simulink model "WF_onshore"  (R2024a)
settings: Solver=VariableStepAuto  StartTime=0  StopTime=0.9  RelTol=1e-3
values from neighbouring files (symbols this model uses):
  cvtr = initialize_NR_VSC_GF(cvtr)    [NR_steadystate_VSC_GF.m]    (also in WF_onshore_SSO_GFL.m = setfield(cvtr,'parameters', p_vary.name,p_vary.val(i)); WF_physical_param_offshore_supersynchronous.m = setfield(cvtr,'parameters', p_vary.name,p_vary.val(i)); WF_physical_param_onshore_SSO_020625.m = setfield(cvtr,'parameters', p_vary.name,p_vary.val(i)); impedance_WT_blackbox.m = base_values(cvtr))
  cvtr1 = cvtr_agg    [WF_physical_param_onshore_SSO_020625.m]
  enable_pll = 1    [impedance_WT_agg.m]    (also in initialize_WT_agg.m; initialize_WT_default_gfl.m; initialize_WT_default_offshore_super.m)
  f1 = 50    [WF_onshore_SSO_GFL.m]    (also in WF_physical_param_offshore_supersynchronous.m; WF_physical_param_onshore_SSO_020625.m; initialize_params_agg.m)
  i = 1    [WF_physical_param_offshore_supersynchronous.m]    (also in WF_physical_param_onshore_SSO_020625.m)
  L = inv(R)    [participation_factors_VSC_GF.m]
  l_OH = 0.2    [WF_onshore_SSO_GFL.m]    (also in WF_physical_param_offshore_supersynchronous.m = 0.1; WF_physical_param_onshore_SSO_020625.m = 0.1; initialize_params_agg.m = 0.1)
  l_tf_wf = tf_params(2,2)    [IM_WF_agg.m]    (also in WF_onshore_SSO_GFL.m = 0.05; WF_physical_param_offshore_supersynchronous.m = 0.05; WF_physical_param_onshore_SSO_020625.m = 0.05; initialize_params_agg.m = 0.05)
  l_tf_wt = tf_params(1,2)    [IM_WF_agg.m]    (also in WF_onshore_SSO_GFL.m = 0.0392; WF_physical_param_offshore_supersynchronous.m = 0.0392; WF_physical_param_onshore_SSO_020625.m = 0.0392; initialize_params_agg.m = 0.0392)
  Lg = p_vary(i)*((Z_b_G/(2*pi*f1)))    [WF_onshore_SSO_GFL.m]    (also in WF_physical_param_offshore_supersynchronous.m; WF_physical_param_onshore_SSO_020625.m; initialize_params_agg.m = 0.1*((Z_b_G/(2*pi*f1))))
  Lg1 = Lg    [WF_physical_param_offshore_supersynchronous.m]    (also in WF_physical_param_onshore_SSO_020625.m)
  Lg2 = Lg    [WF_physical_param_offshore_supersynchronous.m]    (also in WF_physical_param_onshore_SSO_020625.m)
  r_OH = 0.02    [WF_onshore_SSO_GFL.m]    (also in WF_physical_param_offshore_supersynchronous.m = 0.01; WF_physical_param_onshore_SSO_020625.m = 0.01; initialize_params_agg.m)
  r_tf_wf = tf_params(2,1)    [IM_WF_agg.m]    (also in WF_onshore_SSO_GFL.m = 0.005; WF_physical_param_offshore_supersynchronous.m = 0.005; WF_physical_param_onshore_SSO_020625.m = 0.005; initialize_params_agg.m = 0.005)
  r_tf_wt = tf_params(1,1)    [IM_WF_agg.m]    (also in WF_onshore_SSO_GFL.m = 0.0056; WF_physical_param_offshore_supersynchronous.m = 0.0056; WF_physical_param_onshore_SSO_020625.m = 0.0056; initialize_params_agg.m = 0.0056)
  Rg = rg*Z_b_G    [WF_onshore_SSO_GFL.m]    (also in WF_physical_param_offshore_supersynchronous.m; WF_physical_param_onshore_SSO_020625.m; initialize_params_agg.m = 0.01*Z_b_G)
  Sb_WF = (3*1)*5e6    (= 15000000)    [WF_onshore_SSO_GFL.m]    (also in WF_physical_param_offshore_supersynchronous.m; WF_physical_param_onshore_SSO_020625.m; impedance_WT_blackbox.m = n_t*Sb_WT; initialize_params_agg.m = 1000000000)
  Sb_WT = 5e6    (= 5000000)    [IM_WF.m]    (also in WF_onshore_SSO_GFL.m; WF_physical_param_offshore_supersynchronous.m; WF_physical_param_onshore_SSO_020625.m; initialize_params_agg.m)
  selector_current_reference = 3    [impedance_WT_agg.m]    (also in initialize_WT_agg.m; initialize_WT_default_gfl.m; initialize_WT_default_offshore_super.m)
  selector_omega_reference = 1    [impedance_WT_agg.m]    (also in initialize_WT_agg.m; initialize_WT_default_gfl.m; initialize_WT_default_offshore_super.m)
  V_coll = 33e3    (= 33000)    [WF_onshore_SSO_GFL.m]    (also in WF_physical_param_offshore_supersynchronous.m; WF_physical_param_onshore_SSO_020625.m; initialize_params_agg.m)
  V_trans = 220e3    (= 220000)    [WF_onshore_SSO_GFL.m]    (also in WF_physical_param_offshore_supersynchronous.m; WF_physical_param_onshore_SSO_020625.m; initialize_params_agg.m)
  Z_b_G = (V_trans/sqrt(3/2))^2/Sb_WF    [WF_onshore_SSO_GFL.m]    (also in WF_physical_param_offshore_supersynchronous.m = (V_b_trans)^2/Sb_WF; WF_physical_param_onshore_SSO_020625.m = (V_b_trans)^2/Sb_WF; initialize_params_agg.m = (V_b_trans)^2/Sb_WF)
undefined symbols (not defined in the file or in its folder): opts, R
libraries: simulink_extras x104, spsSeriesRLCBranchLib x90, simulink x52, spsThreePhaseVIMeasurementLib x42, spsControlledVoltageSourceLib x42, spsGroundLib x27, spsThreePhaseTransformerTwoWindingsLib x14, powerlib_extras x13, spsVariableInductorLib x6, spsPower3phInstantaneousLib x3, spspowerguiLib x1
(part 8 of 12)

== system WF_onshore/WT_MF12/Control System/Voltage controller DEM ==
  ve : Inport
  vo : Inport  Port=2
  Omegavsm : Inport  Port=3
  ilr0 : Inport  Port=4
  Enable : EnablePort
  Gain : Gain  Gain=cvtr.pu.Omegab/cvtr.parameters.ls
  Gain1 : Gain  Gain=cvtr.pu.Omegab/cvtr.parameters.ls
  Gain2 : Gain  Gain=cvtr.pu.Omegab*cvtr.parameters.rs/cvtr.parameters.ls
  Gain3 : Gain  Gain=1i*cvtr.pu.Omegab
  Product : Product  RndMeth=Zero
  Subsystem : Subsystem
  Subtract : Sum  Inputs=+---
  ilr : Outport
  wires:
  ilr0/1 -> Subsystem/2(x0)
  Subsystem/1(x/s) -> ilr/1, Gain2/1, Product/1
  ve/1 -> Gain/1
  Gain/1 -> Subtract/1
  vo/1 -> Gain1/1
  Gain1/1 -> Subtract/2
  Subtract/1 -> Subsystem/1(x)
  Gain2/1 -> Subtract/3
  Gain3/1 -> Subtract/4
  Product/1 -> Gain3/1
  Omegavsm/1 -> Product/2

== system WF_onshore/WT_MF12/Control System/Voltage controller QSEM ==
  ve : Inport
  vo : Inport  Port=2
  Omegavsm : Inport  Port=3
  Enable : EnablePort
  Constant : Constant  Value=cvtr.pu.Omegab*cvtr.parameters.rs/cvtr.parameters.ls
  Demux : Demux  Outputs=2
  Demux1 : Demux  Outputs=2
  Divide : Product  Inputs=*/
  Gain : Gain  Gain=cvtr.pu.Omegab/cvtr.parameters.ls
  Gain1 : Gain  Gain=cvtr.pu.Omegab/cvtr.parameters.ls
  Gain3 : Gain  Gain=1i*cvtr.pu.Omegab
  Mux : Mux  Inputs=2
  Subsystem2 : Subsystem
  Subsystem3 : Subsystem
  Subtract : Sum  Inputs=+-
  Subtract1 : Sum
  Terminator : Terminator
  Terminator1 : Terminator
  Transfer Fcn (with initial outputs) : simulink_extras/Additional Linear/Transfer Fcn (with initial outputs)  N=[cvtr.parameters.Omegavo]  D="[1  cvtr.parameters.Omegavo]"  Y0=cvtr.ss.vomd0  U0=cvtr.ss.vomd0
  Transfer Fcn (with initial outputs)1 : simulink_extras/Additional Linear/Transfer Fcn (with initial outputs)  N=[cvtr.parameters.Omegavo]  D="[1  cvtr.parameters.Omegavo]"  Y0=cvtr.ss.vomq0  U0=cvtr.ss.vomq0
  ilr : Outport
  wires:
  Transfer Fcn (with initial outputs)1/1 -> Mux/2
  Demux/2 -> Transfer Fcn (with initial outputs)1/1
  Demux/1 -> Transfer Fcn (with initial outputs)/1
  Demux1/2 -> Terminator1/1  "vomq?"
  Demux1/1 -> Terminator/1  "vomd?"
  Subsystem3/1(x_d+ix_q) -> Gain1/1
  Mux/1 -> Subsystem3/1(x_dq), Demux1/1
  Transfer Fcn (with initial outputs)/1 -> Mux/1
  Subsystem2/1(x_dq) -> Demux/1
  vo/1 -> Subsystem2/1(x_d+ix_q)
  Subtract1/1 -> Divide/2
  Divide/1 -> ilr/1
  Constant/1 -> Subtract1/1
  Subtract/1 -> Divide/1
  ve/1 -> Gain/1
  Gain/1 -> Subtract/1
  Gain1/1 -> Subtract/2
  Gain3/1 -> Subtract1/2
  Omegavsm/1 -> Gain3/1

== system WF_onshore/WT_MF12/Control System/Voltage controller VCVSM ==
  note: PI regulator
  note: Decoupling term
  note: Feedforward
  note: Voltage controller
  vo : Inport
  Omega : Inport  Port=2
  io : Inport  Port=3
  ve : Inport  Port=4
  Enable : EnablePort
  Gain : Gain  Gain=cvtr.parameters.kpv
  Gain1 : Gain  Gain=cvtr.parameters.rs
  Gain2 : Gain  Gain=cvtr.parameters.kiv
  Gain3 : Gain  Gain=1i*cvtr.parameters.cf
  Gain4 : Gain  Gain=cvtr.parameters.kffi
  Gain5 : Gain  Gain=1i*cvtr.parameters.ls
  Omega1 : InportShadow  Port=2
  Product : Product  RndMeth=Zero
  Product1 : Product
  Subsystem : Subsystem
  Subtract : Sum  Inputs=+--
  Subtract1 : Sum  Inputs=|++
  Subtract2 : Sum  Inputs=|++
  Subtract3 : Sum  Inputs=|+-
  Subtract5 : Sum  Inputs=|++
  delta1 : Constant  Value=cvtr.ss.Xi0
  io1 : InportShadow  Port=3
  vo1 : InportShadow
  ilr : Outport
  wires:
  Gain1/1 -> Subtract/2
  ve/1 -> Subtract/1
  Product1/1 -> Gain5/1
  Gain5/1 -> Subtract/3
  Omega1/1 -> Product1/2
  io1/1 -> Product1/1, Gain1/1
  Subtract5/1 -> ilr/1
  Subtract2/1 -> Subtract5/1
  Subtract1/1 -> Subtract2/1
  vo1/1 -> Product/1
  Subsystem/1(x/s) -> Gain2/1  "Xi"
  vo/1 -> Subtract3/2
  Subtract3/1 -> Subsystem/1(x), Gain/1
  delta1/1 -> Subsystem/2(x0)
  Gain4/1 -> Subtract5/2
  io/1 -> Gain4/1
  Omega/1 -> Product/2
  Product/1 -> Gain3/1
  Gain3/1 -> Subtract2/2
  Gain2/1 -> Subtract1/2
  Gain/1 -> Subtract1/1
  Subtract/1 -> Subtract3/1  "vor"

== system WF_onshore/WT_MF12/Control System/q droop1 ==
  q : Inport
  qref : Inport  Port=2
  vref : Inport  Port=3
  Gain3 : Gain  Gain=cvtr.parameters.kdrpq
  Subtract : Sum
  Subtract3 : Sum  Inputs=-+
  Transfer Fcn (with initial outputs) : simulink_extras/Additional Linear/Transfer Fcn (with initial outputs)  N=[cvtr.parameters.Omegaqf]  D="[1  cvtr.parameters.Omegaqf]"  Y0=cvtr.ss.q0  U0=cvtr.ss.q0
  ve : Outport
  qm : Outport  Port=2
  wires:
  q/1 -> Transfer Fcn (with initial outputs)/1
  Subtract/1 -> ve/1
  Gain3/1 -> Subtract/1
  Subtract3/1 -> Gain3/1
  Transfer Fcn (with initial outputs)/1 -> qm/1, Subtract3/1
  qref/1 -> Subtract3/2
  vref/1 -> Subtract/2

== system WF_onshore/WT_MF12/Transformations (pu and dq)/Park ==
  x_abc : Inport
  delta : Inport  Port=2
  Demux1 : Demux  Outputs=3
  Fcn : Fcn  Expr=2/3*(cos(u(4))*u(1)+cos(u(4)-2/3*pi)*u(2)+cos(u(4)+2/3*pi)*u(3))
  Fcn1 : Fcn  Expr=-2/3*(sin(u(4))*u(1)+sin(u(4)-2/3*pi)*u(2)+sin(u(4)+2/3*pi)*u(3))
  Mux : Mux
  Mux1 : Mux  Inputs=2
  x_dq : Outport
  wires:
  Mux1/1 -> x_dq/1
  Fcn1/1 -> Mux1/2
  Fcn/1 -> Mux1/1
  Mux/1 -> Fcn1/1, Fcn/1
  delta/1 -> Mux/4
  x_abc/1 -> Demux1/1
  Demux1/3 -> Mux/3
  Demux1/2 -> Mux/2
  Demux1/1 -> Mux/1

== system WF_onshore/WT_MF12/Transformations (pu and dq)/Park1 ==
  x_abc : Inport
  delta : Inport  Port=2
  Demux1 : Demux  Outputs=3
  Fcn : Fcn  Expr=2/3*(cos(u(4))*u(1)+cos(u(4)-2/3*pi)*u(2)+cos(u(4)+2/3*pi)*u(3))
  Fcn1 : Fcn  Expr=-2/3*(sin(u(4))*u(1)+sin(u(4)-2/3*pi)*u(2)+sin(u(4)+2/3*pi)*u(3))
  Mux : Mux
  Mux1 : Mux  Inputs=2
  x_dq : Outport
  wires:
  Demux1/1 -> Mux/1
  Demux1/2 -> Mux/2
  Demux1/3 -> Mux/3
  x_abc/1 -> Demux1/1
  delta/1 -> Mux/4
  Mux/1 -> Fcn/1, Fcn1/1
  Fcn/1 -> Mux1/1
  Fcn1/1 -> Mux1/2
  Mux1/1 -> x_dq/1

== system WF_onshore/WT_MF12/Transformations (pu and dq)/Park2 ==
  x_abc : Inport
  delta : Inport  Port=2
  Demux1 : Demux  Outputs=3
  Fcn : Fcn  Expr=2/3*(cos(u(4))*u(1)+cos(u(4)-2/3*pi)*u(2)+cos(u(4)+2/3*pi)*u(3))
  Fcn1 : Fcn  Expr=-2/3*(sin(u(4))*u(1)+sin(u(4)-2/3*pi)*u(2)+sin(u(4)+2/3*pi)*u(3))
  Mux : Mux
  Mux1 : Mux  Inputs=2
  x_dq : Outport
  wires:
  Demux1/1 -> Mux/1
  Demux1/2 -> Mux/2
  Demux1/3 -> Mux/3
  x_abc/1 -> Demux1/1
  delta/1 -> Mux/4
  Mux/1 -> Fcn/1, Fcn1/1
  Fcn/1 -> Mux1/1
  Fcn1/1 -> Mux1/2
  Mux1/1 -> x_dq/1

== system WF_onshore/WT_MF12/Transformations (pu and dq)/Park4 ==
  x_abc : Inport
  delta : Inport  Port=2
  Demux1 : Demux  Outputs=3
  Fcn : Fcn  Expr=2/3*(cos(u(4))*u(1)+cos(u(4)-2/3*pi)*u(2)+cos(u(4)+2/3*pi)*u(3))
  Fcn1 : Fcn  Expr=-2/3*(sin(u(4))*u(1)+sin(u(4)-2/3*pi)*u(2)+sin(u(4)+2/3*pi)*u(3))
  Mux : Mux
  Mux1 : Mux  Inputs=2
  x_dq : Outport
  wires:
  Demux1/1 -> Mux/1
  Demux1/2 -> Mux/2
  Demux1/3 -> Mux/3
  x_abc/1 -> Demux1/1
  delta/1 -> Mux/4
  Mux/1 -> Fcn/1, Fcn1/1
  Fcn/1 -> Mux1/1
  Fcn1/1 -> Mux1/2
  Mux1/1 -> x_dq/1

== system WF_onshore/WT_MF12/Transformations (pu and dq)/Subsystem2 ==
  x_dq : Inport
  Demux : Demux  Outputs=2
  Real-Imag to Complex : RealImagToComplex
  x_d+ix_q : Outport
  wires:
  Real-Imag to Complex/1 -> x_d+ix_q/1
  x_dq/1 -> Demux/1
  Demux/2 -> Real-Imag to Complex/2
  Demux/1 -> Real-Imag to Complex/1

== system WF_onshore/WT_MF12/Transformations (pu and dq)/Subsystem3 ==
  x_dq : Inport
  Demux : Demux  Outputs=2
  Real-Imag to Complex : RealImagToComplex
  x_d+ix_q : Outport
  wires:
  Real-Imag to Complex/1 -> x_d+ix_q/1
  x_dq/1 -> Demux/1
  Demux/2 -> Real-Imag to Complex/2
  Demux/1 -> Real-Imag to Complex/1

== system WF_onshore/WT_MF12/Transformations (pu and dq)/Subsystem4 ==
  x_dq : Inport
  Demux : Demux  Outputs=2
  Real-Imag to Complex : RealImagToComplex
  x_d+ix_q : Outport
  wires:
  Real-Imag to Complex/1 -> x_d+ix_q/1
  x_dq/1 -> Demux/1
  Demux/2 -> Real-Imag to Complex/2
  Demux/1 -> Real-Imag to Complex/1

== system WF_onshore/WT_MF12/Transformations (pu and dq)/Subsystem7 ==
  x_dq : Inport
  Demux : Demux  Outputs=2
  Real-Imag to Complex : RealImagToComplex
  x_d+ix_q : Outport
  wires:
  Demux/1 -> Real-Imag to Complex/1
  Demux/2 -> Real-Imag to Complex/2
  x_dq/1 -> Demux/1
  Real-Imag to Complex/1 -> x_d+ix_q/1

== system WF_onshore/WT_MF14/Control System/Current controller ==
  note: Active damping
  note: Feedforward
  note: Decoupling term
  note: PI regulator
  ilr : Inport
  il : Inport  Port=2
  Omega : Inport  Port=3
  vo : Inport  Port=4
  Gain : Gain  Gain=cvtr.parameters.kpc
  Gain1 : Gain
  Gain2 : Gain  Gain=cvtr.parameters.kic
  Gain3 : Gain  Gain=1i*cvtr.parameters.lf
  Gain4 : Gain  Gain=cvtr.parameters.kffv
  Gain5 : Gain  Gain=cvtr.parameters.kad
  Product : Product  RndMeth=Zero
  Scope : Scope  Commented=on  NumInputPorts=2
  Subsystem : Subsystem
  Subsystem1 : Subsystem  mask{Omega=cvtr.parameters.Omegaad, xd0=cvtr.ss.Phid0, xq0=cvtr.ss.Phiq0}
  Subtract1 : Sum  Inputs=|++
  Subtract2 : Sum  Inputs=|++
  Subtract3 : Sum  Inputs=|+-
  Subtract4 : Sum  Inputs=|+-
  Subtract5 : Sum  Inputs=|++
  Subtract6 : Sum  Inputs=|+-
  delta1 : Constant  Value=cvtr.ss.Gamma0
  il1 : InportShadow  Port=2
  vo1 : InportShadow  Port=4
  vir : Outport
  wires:
  Gain2/1 -> Subtract1/2
  Gain3/1 -> Subtract2/2
  Product/1 -> Gain3/1
  Omega/1 -> Product/2
  vo/1 -> Gain4/1
  Gain4/1 -> Subtract5/2
  Gain5/1 -> Subtract6/2
  Subtract4/1 -> Gain5/1
  delta1/1 -> Subsystem/2(x0)
  il/1 -> Scope/2, Subtract3/2
  Subsystem/1(x/s) -> Gain2/1  "Gamma"
  il1/1 -> Product/1
  Subtract1/1 -> Subtract2/1
  vo1/1 -> Subsystem1/1(in), Subtract4/1
  Subsystem1/1(out) -> Subtract4/2
  Subtract2/1 -> Subtract5/1
  Subtract5/1 -> Subtract6/1
  Gain/1 -> Subtract1/1
  Subtract6/1 -> Gain1/1
  Gain1/1 -> vir/1
  Subtract3/1 -> Subsystem/1(x), Gain/1
  ilr/1 -> Scope/1, Subtract3/1

== system WF_onshore/WT_MF14/Control System/GFL state space ==
  io : Inport
  omega : Inport  Port=2
  il : Inport  Port=3
  vo : Inport  Port=4
  Input : Inport  Port=5
  " " : Scope
  " l" : Scope
  Add{1..6,9} (7 alike) : Sum
  Add7 : Sum  Inputs=-+
  Add8 : Sum  Inputs=-+
  Demux{1..4} (4 alike) : Demux  Outputs=2
  Gain1 : Gain
  Mux{1..3,5,8} (5 alike) : Mux  Inputs=2
  Mux4 : Mux  Inputs=5
  Omegapll : Scope
  Product{,1..7} (8 alike) : Product
  Scope : Scope  NumInputPorts=2
  Scope1 : Scope  NumInputPorts=2
  Selector1 : Selector  IndexOptions=Index vector (dialog)  Indices=15  OutputSizes=1
  Selector2 : Selector  IndexOptions=Index vector (dialog)  Indices=[1,2]  OutputSizes=1
  Selector3 : Selector  IndexOptions=Index vector (dialog)  Indices=[3,4]  OutputSizes=1
  Selector4 : Selector  IndexOptions=Index vector (dialog)  Indices=16  OutputSizes=1
  Selector5 : Selector  IndexOptions=Index vector (dialog)  Indices=[5,6]  OutputSizes=1
  State-Space : StateSpace  A=cvtr.A  B=cvtr.B  C=eye(size(cvtr.A))  D=zeros(size(cvtr.B))  InitialCondition=0
  Subsystem5 : Subsystem
  Subsystem8 : Subsystem
  Subsystem9 : Subsystem
  Theta : Scope
  delta1 : Constant  Value=[real(cvtr.ss.il0),imag(cvtr.ss.il0)]
  delta16 : Constant  Value=[real(cvtr.ss.io0),imag(cvtr.ss.io0)]
  delta2 : Constant  Value=[real(cvtr.ss.vo0),imag(cvtr.ss.vo0)]
  delta5 : Constant  Value=cvtr.ss.DeltaThetapll0
  delta6 : Constant  Value=cvtr.ss.Omegapll0
  v : Scope
  wires:
  io/1 -> Subsystem9/1(x_d+ix_q)
  delta6/1 -> Add1/2
  Add5/1 -> Demux1/1, Mux8/2
  Mux1/1 -> Omegapll/1
  Mux2/1 -> " l"/1
  Mux3/1 -> v/1
  omega/1 -> Mux1/1
  delta1/1 -> Add2/2
  Add3/1 -> Demux2/1, Mux3/2
  delta2/1 -> Add3/2
  Selector5/1 -> Gain1/1
  Mux8/1 -> " "/1
  Add1/1 -> Mux1/2
  vo/1 -> Subsystem8/1(x_d+ix_q)
  il/1 -> Subsystem5/1(x_d+ix_q)
  Add2/1 -> Mux2/2
  delta16/1 -> Add5/2
  Selector2/1 -> Add2/1
  Selector1/1 -> Add1/1
  State-Space/1 -> Selector5/1, Selector1/1, Selector3/1, Selector4/1, Selector2/1
  Subsystem5/1(x_dq) -> Mux2/1
  Mux4/1 -> State-Space/1
  Demux1/1 -> Product5/2, Product/1  "id"
  Demux2/1 -> Product4/1, Product/2  "vd"
  Demux1/2 -> Product4/2, Product1/1  "iq"
  Demux2/2 -> Product5/1, Product1/2  "vq"
  Product/1 -> Add4/1
  Product1/1 -> Add4/2
  Add4/1 -> Scope/1  "p_ss"
  Product3/1 -> Add6/2
  Product2/1 -> Add6/1
  Demux4/2 -> Product7/1, Product3/2  "vq"
  Demux3/2 -> Product6/2, Product3/1  "iq"
  Demux4/1 -> Product2/2, Product6/1  "vd"
  Demux3/1 -> Product7/2, Product2/1  "id"
  Subsystem8/1(x_dq) -> Demux4/1, Mux3/1
  Subsystem9/1(x_dq) -> Demux3/1, Mux8/1
  Add6/1 -> Scope/2  "p_dq"
  Product4/1 -> Add7/1
  Product5/1 -> Add7/2
  Add7/1 -> Scope1/1  "q_ss"
  Add8/1 -> Scope1/2  "q"
  Product7/1 -> Add8/2
  Product6/1 -> Add8/1
  [d_input] -> Mux4/5
  Gain1/1 -> Add5/1
  Selector3/1 -> Add3/1
  Mux5/1 -> Theta/1
  Add9/1 -> Mux5/2
  delta5/1 -> Add9/2
  Selector4/1 -> Add9/1
  Input/1 -> Mux5/1
  [dvnq] -> Mux4/4
  [dvnd] -> Mux4/3
  [d_pref] -> Mux4/1
  [d_qref] -> Mux4/2

== system WF_onshore/WT_MF14/Control System/GFM State Space model ==
  io : Inport
  omega : Inport  Port=2
  il : Inport  Port=3
  vo : Inport  Port=4
  In5 : Inport  Port=5
  " " : Scope
  " l" : Scope
  Add{1..3,5,9} (5 alike) : Sum
  Gain : Gain  Gain=-1
  Gain1 : Gain
  Mux{1..3,5,8} (5 alike) : Mux  Inputs=2
  Mux4 : Mux  Inputs=7
  Omegapll : Scope
  Selector1 : Selector  IndexOptions=Index vector (dialog)  Indices=12  OutputSizes=1
  Selector2 : Selector  IndexOptions=Index vector (dialog)  Indices=[1,2]  OutputSizes=1
  Selector3 : Selector  IndexOptions=Index vector (dialog)  Indices=[3,4]  OutputSizes=1
  Selector4 : Selector  IndexOptions=Index vector (dialog)  Indices=13  OutputSizes=1
  Selector5 : Selector  IndexOptions=Index vector (dialog)  Indices=[5,6]  OutputSizes=1
  State-Space : StateSpace  A=cvtr.A  B=cvtr.B  C=eye(size(cvtr.A))  D=zeros(size(cvtr.B))  InitialCondition=0
  Subsystem5 : Subsystem
  Subsystem8 : Subsystem
  Subsystem9 : Subsystem
  Theta : Scope
  delta1 : Constant  Value=[real(cvtr.ss.il0),imag(cvtr.ss.il0)]
  delta16 : Constant  Value=[real(cvtr.ss.io0),imag(cvtr.ss.io0)]
  delta2 : Constant  Value=[real(cvtr.ss.vo0),imag(cvtr.ss.vo0)]
  delta5 : Constant  Value=cvtr.ss.DeltaThetavsm0
  delta6 : Constant  Value=cvtr.ss.Omegapll0
  v : Scope
  wires:
  [dvnd] -> Mux4/3
  [dvnq] -> Mux4/4
  Selector3/1 -> Add3/1
  Gain1/1 -> Add5/1
  [d_input] -> Mux4/7
  Subsystem9/1(x_dq) -> Mux8/1
  Subsystem8/1(x_dq) -> Mux3/1
  Mux4/1 -> State-Space/1
  Subsystem5/1(x_dq) -> Mux2/1
  State-Space/1 -> Selector2/1, Selector3/1, Selector4/1, Selector1/1, Selector5/1
  Selector1/1 -> Add1/1
  Selector2/1 -> Add2/1
  delta16/1 -> Add5/2
  Add2/1 -> Mux2/2
  il/1 -> Subsystem5/1(x_d+ix_q)
  vo/1 -> Subsystem8/1(x_d+ix_q)
  Add1/1 -> Mux1/2
  Mux8/1 -> " "/1
  Selector5/1 -> Gain1/1
  delta2/1 -> Add3/2
  Add3/1 -> Mux3/2
  delta1/1 -> Add2/2
  omega/1 -> Mux1/1
  Mux3/1 -> v/1
  Mux2/1 -> " l"/1
  Mux1/1 -> Omegapll/1
  Add5/1 -> Mux8/2
  delta6/1 -> Add1/2
  io/1 -> Subsystem9/1(x_d+ix_q)
  [d_pref] -> Mux4/1
  [d_qref] -> Mux4/2
  [d_Vref] -> Mux4/5
  [d_Oref] -> Mux4/6
  In5/1 -> Gain/1
  Selector4/1 -> Add9/1
  Add9/1 -> Mux5/2
  Mux5/1 -> Theta/1
  delta5/1 -> Add9/2
  Gain/1 -> Mux5/1

== system WF_onshore/WT_MF14/Control System/Mechanical1 ==
  p : Inport
  pref : Inport  Port=2
  DeltaThetavsm0 : Inport  Port=3
  Omegavsm0 : Inport  Port=4
  Omegaref : Inport  Port=5
  Omegapll : Inport  Port=6
  Constant : Constant  Value=enable_pll
  Gain : Gain  Gain=1/cvtr.parameters.ta
  Gain1 : Gain  Gain=cvtr.parameters.kd
  Gain2 : Gain  Gain=cvtr.parameters.kdrpOmega
  Gain3 : Gain  Gain=cvtr.pu.Omegab
  Integrator1 : Integrator  InitialConditionSource=external
  Integrator2 : Integrator  InitialConditionSource=external
  Subtract : Sum  Inputs=-+--
  Subtract1 : Sum  Inputs=-+
  Subtract2 : Sum  Inputs=-+
  Switch : Switch  Criteria=u2 > Threshold  SaturateOnIntegerOverflow=off  InputSameDT=off
  Transfer Fcn (with initial outputs) : simulink_extras/Additional Linear/Transfer Fcn (with initial outputs)  N=[cvtr.parameters.Omegadf]  D="[1  cvtr.parameters.Omegadf]"  Y0=cvtr.ss.Kappa0  U0=cvtr.ss.Kappa0
  Thetavsm : Outport
  Omegavsm : Outport  Port=2
  wires:
  DeltaThetavsm0/1 -> Integrator1/2
  p/1 -> Subtract/1
  pref/1 -> Subtract/2
  Subtract/1 -> Gain/1
  Gain1/1 -> Subtract/3
  Subtract1/1 -> Gain1/1
  Omegavsm0/1 -> Integrator2/2
  Gain/1 -> Integrator2/1
  Omegaref/1 -> Subtract2/1
  Subtract2/1 -> Gain2/1
  Gain2/1 -> Subtract/4
  Gain3/1 -> Integrator1/1
  Omegapll/1 -> Switch/1
  Constant/1 -> Switch/2
  Transfer Fcn (with initial outputs)/1 -> Switch/3
  Integrator2/1 -> Gain3/1, Transfer Fcn (with initial outputs)/1, Subtract2/2, Subtract1/2, Omegavsm/1
  Switch/1 -> Subtract1/1
  Integrator1/1 -> Thetavsm/1

== system WF_onshore/WT_MF14/Control System/PLL1 ==
  note: DeltaOmegapll
  vo : Inport
  Add : Sum
  Add3 : Sum
  Constant : Constant  Value=cvtr.ss.Epsilonpll0
  Constant1 : Constant  Value=cvtr.ss.DeltaThetapll0
  Constant3 : Constant  Value=-cvtr.ss.DeltaThetapll0
  Constant4 : Constant  Value=cvtr.parameters.Omegan
  Demux : Demux  Outputs=2
  Demux1 : Demux  Outputs=2
  Gain : Gain  Gain=cvtr.parameters.kppll
  Gain1 : Gain  Gain=cvtr.pu.Omegab
  Gain2 : Gain  Gain=cvtr.parameters.kipll
  Integrator1 : Integrator  InitialConditionSource=external
  Integrator2 : Integrator  InitialConditionSource=external
  Multiport Switch1 : MultiPortSwitch  DataPortOrder=Zero-based contiguous  Inputs=2  zeroidx=on  SaturateOnIntegerOverflow=off  InputSameDT=off
  Mux : Mux  Inputs=2
  Scope : Scope  Commented=on
  Subsystem1 : Subsystem
  Subsystem3 : Subsystem
  Terminator : Terminator
  Terminator1 : Terminator
  Transfer Fcn (with initial outputs) : simulink_extras/Additional Linear/Transfer Fcn (with initial outputs)  N=[cvtr.parameters.Omegalppll]  D="[1  cvtr.parameters.Omegalppll]"  Y0=real(cvtr.ss.vpll0)  U0=real(cvtr.ss.vpll0)
  Transfer Fcn (with initial outputs)1 : simulink_extras/Additional Linear/Transfer Fcn (with initial outputs)  N=[cvtr.parameters.Omegalppll]  D="[1  cvtr.parameters.Omegalppll]"  Y0=imag(cvtr.ss.vpll0)  U0=imag(cvtr.ss.vpll0)
  Trigonometric Function : Trigonometry  Operator=atan2
  delta6 : Constant  Value=selector_omega_reference
  Omegapll : Outport
  vpll : Outport  Port=2
  Thetapll : Outport  Port=3
  wires:
  vo/1 -> Subsystem1/1(x_d+ix_q)
  Subsystem1/1(x_dq) -> Demux/1
  Transfer Fcn (with initial outputs)1/1 -> Trigonometric Function/1, Mux/2
  Trigonometric Function/1 -> Integrator2/1, Gain/1
  Gain/1 -> Add/1
  Constant/1 -> Integrator2/2
  Gain2/1 -> Add/2
  Add/1 -> Add3/2
  Subsystem3/1(x_d+ix_q) -> vpll/1
  Add3/1 -> Scope/1, Omegapll/1, Gain1/1
  Constant4/1 -> Add3/1
  Gain1/1 -> Integrator1/1
  Mux/1 -> Demux1/1, Subsystem3/1(x_dq)
  Demux1/2 -> Terminator1/1  "vpll_q"
  Demux1/1 -> Terminator/1  "vpll_d"
  Demux/1 -> Transfer Fcn (with initial outputs)/1
  Transfer Fcn (with initial outputs)/1 -> Mux/1, Trigonometric Function/2
  Integrator2/1 -> Gain2/1
  Integrator1/1 -> Thetapll/1
  Constant3/1 -> Multiport Switch1/3
  delta6/1 -> Multiport Switch1/1
  Constant1/1 -> Multiport Switch1/2
  Multiport Switch1/1 -> Integrator1/2
  Demux/2 -> Transfer Fcn (with initial outputs)1/1

== system WF_onshore/WT_MF14/Control System/PQ controller ==
  note: PI regulator
  note: PI regulator
  pref : Inport
  p : Inport  Port=2
  qref : Inport  Port=3
  q : Inport  Port=4
  Enable : EnablePort
  Gain : Gain  Gain=cvtr.parameters.kpp
  Gain1 : Gain  Gain=cvtr.parameters.kpq
  Gain2 : Gain  Gain=cvtr.parameters.kip
  Gain3 : Gain  Gain=cvtr.parameters.kiq
  Gain4 : Gain
  Gain5 : Gain  Gain=-1
  Integrator1 : Integrator  InitialConditionSource=external
  Integrator2 : Integrator  InitialConditionSource=external
  Mux : Mux  Inputs=2
  Subsystem3 : Subsystem
  Subtract1 : Sum  Inputs=|++
  Subtract2 : Sum  Inputs=|++
  Subtract3 : Sum  Inputs=|+-
  Subtract4 : Sum  Inputs=|+-
  delta1 : Constant  Value=cvtr.ss.GammaSd0
  delta2 : Constant  Value=cvtr.ss.GammaSq0
  ir : Outport
  wires:
  Gain/1 -> Subtract1/1
  Integrator1/1 -> Gain2/1
  p/1 -> Subtract3/2
  Subtract3/1 -> Integrator1/1, Gain/1
  delta1/1 -> Integrator1/2
  Gain2/1 -> Subtract1/2
  pref/1 -> Subtract3/1
  qref/1 -> Subtract4/1
  Gain3/1 -> Subtract2/2
  delta2/1 -> Integrator2/2
  Subtract4/1 -> Integrator2/1, Gain1/1
  q/1 -> Subtract4/2
  Integrator2/1 -> Gain3/1
  Gain1/1 -> Subtract2/1
  Mux/1 -> Subsystem3/1(x_dq)
  Subtract1/1 -> Gain4/1
  Subtract2/1 -> Gain5/1
  Subsystem3/1(x_d+ix_q) -> ir/1
  Gain5/1 -> Mux/2
  Gain4/1 -> Mux/1

== system WF_onshore/WT_MF14/Control System/Voltage controller DEM ==
  ve : Inport
  vo : Inport  Port=2
  Omegavsm : Inport  Port=3
  ilr0 : Inport  Port=4
  Enable : EnablePort
  Gain : Gain  Gain=cvtr.pu.Omegab/cvtr.parameters.ls
  Gain1 : Gain  Gain=cvtr.pu.Omegab/cvtr.parameters.ls
  Gain2 : Gain  Gain=cvtr.pu.Omegab*cvtr.parameters.rs/cvtr.parameters.ls
  Gain3 : Gain  Gain=1i*cvtr.pu.Omegab
  Product : Product  RndMeth=Zero
  Subsystem : Subsystem
  Subtract : Sum  Inputs=+---
  ilr : Outport
  wires:
  Omegavsm/1 -> Product/2
  Product/1 -> Gain3/1
  Gain3/1 -> Subtract/4
  Gain2/1 -> Subtract/3
  Subtract/1 -> Subsystem/1(x)
  Gain1/1 -> Subtract/2
  vo/1 -> Gain1/1
  Gain/1 -> Subtract/1
  ve/1 -> Gain/1
  Subsystem/1(x/s) -> Product/1, Gain2/1, ilr/1
  ilr0/1 -> Subsystem/2(x0)

== system WF_onshore/WT_MF14/Control System/Voltage controller QSEM ==
  ve : Inport
  vo : Inport  Port=2
  Omegavsm : Inport  Port=3
  Enable : EnablePort
  Constant : Constant  Value=cvtr.pu.Omegab*cvtr.parameters.rs/cvtr.parameters.ls
  Demux : Demux  Outputs=2
  Demux1 : Demux  Outputs=2
  Divide : Product  Inputs=*/
  Gain : Gain  Gain=cvtr.pu.Omegab/cvtr.parameters.ls
  Gain1 : Gain  Gain=cvtr.pu.Omegab/cvtr.parameters.ls
  Gain3 : Gain  Gain=1i*cvtr.pu.Omegab
  Mux : Mux  Inputs=2
  Subsystem2 : Subsystem
  Subsystem3 : Subsystem
  Subtract : Sum  Inputs=+-
  Subtract1 : Sum
  Terminator : Terminator
  Terminator1 : Terminator
  Transfer Fcn (with initial outputs) : simulink_extras/Additional Linear/Transfer Fcn (with initial outputs)  N=[cvtr.parameters.Omegavo]  D="[1  cvtr.parameters.Omegavo]"  Y0=cvtr.ss.vomd0  U0=cvtr.ss.vomd0
  Transfer Fcn (with initial outputs)1 : simulink_extras/Additional Linear/Transfer Fcn (with initial outputs)  N=[cvtr.parameters.Omegavo]  D="[1  cvtr.parameters.Omegavo]"  Y0=cvtr.ss.vomq0  U0=cvtr.ss.vomq0
  ilr : Outport
  wires:
  Omegavsm/1 -> Gain3/1
  Gain3/1 -> Subtract1/2
  Gain1/1 -> Subtract/2
  Gain/1 -> Subtract/1
  ve/1 -> Gain/1
  Subtract/1 -> Divide/1
  Constant/1 -> Subtract1/1
  Divide/1 -> ilr/1
  Subtract1/1 -> Divide/2
  vo/1 -> Subsystem2/1(x_d+ix_q)
  Subsystem2/1(x_dq) -> Demux/1
  Transfer Fcn (with initial outputs)/1 -> Mux/1
  Mux/1 -> Demux1/1, Subsystem3/1(x_dq)
  Subsystem3/1(x_d+ix_q) -> Gain1/1
  Demux1/1 -> Terminator/1  "vomd?"
  Demux1/2 -> Terminator1/1  "vomq?"
  Demux/1 -> Transfer Fcn (with initial outputs)/1
  Demux/2 -> Transfer Fcn (with initial outputs)1/1
  Transfer Fcn (with initial outputs)1/1 -> Mux/2

== system WF_onshore/WT_MF14/Control System/Voltage controller VCVSM ==
  note: Voltage controller
  note: Feedforward
  note: Decoupling term
  note: PI regulator
  vo : Inport
  Omega : Inport  Port=2
  io : Inport  Port=3
  ve : Inport  Port=4
  Enable : EnablePort
  Gain : Gain  Gain=cvtr.parameters.kpv
  Gain1 : Gain  Gain=cvtr.parameters.rs
  Gain2 : Gain  Gain=cvtr.parameters.kiv
  Gain3 : Gain  Gain=1i*cvtr.parameters.cf
  Gain4 : Gain  Gain=cvtr.parameters.kffi
  Gain5 : Gain  Gain=1i*cvtr.parameters.ls
  Omega1 : InportShadow  Port=2
  Product : Product  RndMeth=Zero
  Product1 : Product
  Subsystem : Subsystem
  Subtract : Sum  Inputs=+--
  Subtract1 : Sum  Inputs=|++
  Subtract2 : Sum  Inputs=|++
  Subtract3 : Sum  Inputs=|+-
  Subtract5 : Sum  Inputs=|++
  delta1 : Constant  Value=cvtr.ss.Xi0
  io1 : InportShadow  Port=3
  vo1 : InportShadow
  ilr : Outport
  wires:
  Subtract/1 -> Subtract3/1  "vor"
  Gain/1 -> Subtract1/1
  Gain2/1 -> Subtract1/2
  Gain3/1 -> Subtract2/2
  Product/1 -> Gain3/1
  Omega/1 -> Product/2
  io/1 -> Gain4/1
  Gain4/1 -> Subtract5/2
  delta1/1 -> Subsystem/2(x0)
  Subtract3/1 -> Gain/1, Subsystem/1(x)
  vo/1 -> Subtract3/2
  Subsystem/1(x/s) -> Gain2/1  "Xi"
  vo1/1 -> Product/1
  Subtract1/1 -> Subtract2/1
  Subtract2/1 -> Subtract5/1
  Subtract5/1 -> ilr/1
  io1/1 -> Gain1/1, Product1/1
  Omega1/1 -> Product1/2
  Gain5/1 -> Subtract/3
  Product1/1 -> Gain5/1
  ve/1 -> Subtract/1
  Gain1/1 -> Subtract/2

== system WF_onshore/WT_MF14/Control System/q droop1 ==
  q : Inport
  qref : Inport  Port=2
  vref : Inport  Port=3
  Gain3 : Gain  Gain=cvtr.parameters.kdrpq
  Subtract : Sum
  Subtract3 : Sum  Inputs=-+
  Transfer Fcn (with initial outputs) : simulink_extras/Additional Linear/Transfer Fcn (with initial outputs)  N=[cvtr.parameters.Omegaqf]  D="[1  cvtr.parameters.Omegaqf]"  Y0=cvtr.ss.q0  U0=cvtr.ss.q0
  ve : Outport
  qm : Outport  Port=2
  wires:
  vref/1 -> Subtract/2
  qref/1 -> Subtract3/2
  Transfer Fcn (with initial outputs)/1 -> Subtract3/1, qm/1
  Subtract3/1 -> Gain3/1
  Gain3/1 -> Subtract/1
  Subtract/1 -> ve/1
  q/1 -> Transfer Fcn (with initial outputs)/1

== system WF_onshore/WT_MF14/Transformations (pu and dq)/Park ==
  x_abc : Inport
  delta : Inport  Port=2
  Demux1 : Demux  Outputs=3
  Fcn : Fcn  Expr=2/3*(cos(u(4))*u(1)+cos(u(4)-2/3*pi)*u(2)+cos(u(4)+2/3*pi)*u(3))
  Fcn1 : Fcn  Expr=-2/3*(sin(u(4))*u(1)+sin(u(4)-2/3*pi)*u(2)+sin(u(4)+2/3*pi)*u(3))
  Mux : Mux
  Mux1 : Mux  Inputs=2
  x_dq : Outport
  wires:
  Demux1/1 -> Mux/1
  Demux1/2 -> Mux/2
  Demux1/3 -> Mux/3
  x_abc/1 -> Demux1/1
  delta/1 -> Mux/4
  Mux/1 -> Fcn/1, Fcn1/1
  Fcn/1 -> Mux1/1
  Fcn1/1 -> Mux1/2
  Mux1/1 -> x_dq/1

== system WF_onshore/WT_MF14/Transformations (pu and dq)/Park1 ==
  x_abc : Inport
  delta : Inport  Port=2
  Demux1 : Demux  Outputs=3
  Fcn : Fcn  Expr=2/3*(cos(u(4))*u(1)+cos(u(4)-2/3*pi)*u(2)+cos(u(4)+2/3*pi)*u(3))
  Fcn1 : Fcn  Expr=-2/3*(sin(u(4))*u(1)+sin(u(4)-2/3*pi)*u(2)+sin(u(4)+2/3*pi)*u(3))
  Mux : Mux
  Mux1 : Mux  Inputs=2
  x_dq : Outport
  wires:
  Mux1/1 -> x_dq/1
  Fcn1/1 -> Mux1/2
  Fcn/1 -> Mux1/1
  Mux/1 -> Fcn1/1, Fcn/1
  delta/1 -> Mux/4
  x_abc/1 -> Demux1/1
  Demux1/3 -> Mux/3
  Demux1/2 -> Mux/2
  Demux1/1 -> Mux/1

== system WF_onshore/WT_MF14/Transformations (pu and dq)/Park2 ==
  x_abc : Inport
  delta : Inport  Port=2
  Demux1 : Demux  Outputs=3
  Fcn : Fcn  Expr=2/3*(cos(u(4))*u(1)+cos(u(4)-2/3*pi)*u(2)+cos(u(4)+2/3*pi)*u(3))
  Fcn1 : Fcn  Expr=-2/3*(sin(u(4))*u(1)+sin(u(4)-2/3*pi)*u(2)+sin(u(4)+2/3*pi)*u(3))
  Mux : Mux
  Mux1 : Mux  Inputs=2
  x_dq : Outport
  wires:
  Mux1/1 -> x_dq/1
  Fcn1/1 -> Mux1/2
  Fcn/1 -> Mux1/1
  Mux/1 -> Fcn1/1, Fcn/1
  delta/1 -> Mux/4
  x_abc/1 -> Demux1/1
  Demux1/3 -> Mux/3
  Demux1/2 -> Mux/2
  Demux1/1 -> Mux/1

== system WF_onshore/WT_MF14/Transformations (pu and dq)/Park4 ==
  x_abc : Inport
  delta : Inport  Port=2
  Demux1 : Demux  Outputs=3
  Fcn : Fcn  Expr=2/3*(cos(u(4))*u(1)+cos(u(4)-2/3*pi)*u(2)+cos(u(4)+2/3*pi)*u(3))
  Fcn1 : Fcn  Expr=-2/3*(sin(u(4))*u(1)+sin(u(4)-2/3*pi)*u(2)+sin(u(4)+2/3*pi)*u(3))
  Mux : Mux
  Mux1 : Mux  Inputs=2
  x_dq : Outport
  wires:
  Mux1/1 -> x_dq/1
  Fcn1/1 -> Mux1/2
  Fcn/1 -> Mux1/1
  Mux/1 -> Fcn1/1, Fcn/1
  delta/1 -> Mux/4
  x_abc/1 -> Demux1/1
  Demux1/3 -> Mux/3
  Demux1/2 -> Mux/2
  Demux1/1 -> Mux/1

== system WF_onshore/WT_MF14/Transformations (pu and dq)/Subsystem2 ==
  x_dq : Inport
  Demux : Demux  Outputs=2
  Real-Imag to Complex : RealImagToComplex
  x_d+ix_q : Outport
  wires:
  Demux/1 -> Real-Imag to Complex/1
  Demux/2 -> Real-Imag to Complex/2
  x_dq/1 -> Demux/1
  Real-Imag to Complex/1 -> x_d+ix_q/1

== system WF_onshore/WT_MF14/Transformations (pu and dq)/Subsystem3 ==
  x_dq : Inport
  Demux : Demux  Outputs=2
  Real-Imag to Complex : RealImagToComplex
  x_d+ix_q : Outport
  wires:
  Demux/1 -> Real-Imag to Complex/1
  Demux/2 -> Real-Imag to Complex/2
  x_dq/1 -> Demux/1
  Real-Imag to Complex/1 -> x_d+ix_q/1

== system WF_onshore/WT_MF14/Transformations (pu and dq)/Subsystem4 ==
  x_dq : Inport
  Demux : Demux  Outputs=2
  Real-Imag to Complex : RealImagToComplex
  x_d+ix_q : Outport
  wires:
  Demux/1 -> Real-Imag to Complex/1
  Demux/2 -> Real-Imag to Complex/2
  x_dq/1 -> Demux/1
  Real-Imag to Complex/1 -> x_d+ix_q/1

== system WF_onshore/WT_MF14/Transformations (pu and dq)/Subsystem7 ==
  x_dq : Inport
  Demux : Demux  Outputs=2
  Real-Imag to Complex : RealImagToComplex
  x_d+ix_q : Outport
  wires:
  Real-Imag to Complex/1 -> x_d+ix_q/1
  x_dq/1 -> Demux/1
  Demux/2 -> Real-Imag to Complex/2
  Demux/1 -> Real-Imag to Complex/1

== system WF_onshore/WT_MF2/Control System/Current controller ==
  note: PI regulator
  note: Decoupling term
  note: Feedforward
  note: Active damping
  ilr : Inport
  il : Inport  Port=2
  Omega : Inport  Port=3
  vo : Inport  Port=4
  Gain : Gain  Gain=cvtr.parameters.kpc
  Gain1 : Gain
  Gain2 : Gain  Gain=cvtr.parameters.kic
  Gain3 : Gain  Gain=1i*cvtr.parameters.lf
  Gain4 : Gain  Gain=cvtr.parameters.kffv
  Gain5 : Gain  Gain=cvtr.parameters.kad
  Product : Product  RndMeth=Zero
  Subsystem : Subsystem
  Subsystem1 : Subsystem  mask{Omega=cvtr.parameters.Omegaad, xd0=cvtr.ss.Phid0, xq0=cvtr.ss.Phiq0}
  Subtract1 : Sum  Inputs=|++
  Subtract2 : Sum  Inputs=|++
  Subtract3 : Sum  Inputs=|+-
  Subtract4 : Sum  Inputs=|+-
  Subtract5 : Sum  Inputs=|++
  Subtract6 : Sum  Inputs=|+-
  delta1 : Constant  Value=cvtr.ss.Gamma0
  il1 : InportShadow  Port=2
  vo1 : InportShadow  Port=4
  vir : Outport
  wires:
  ilr/1 -> Subtract3/1
  Subtract3/1 -> Gain/1, Subsystem/1(x)
  Gain1/1 -> vir/1
  Subtract6/1 -> Gain1/1
  Gain/1 -> Subtract1/1
  Subtract5/1 -> Subtract6/1
  Subtract2/1 -> Subtract5/1
  Subsystem1/1(out) -> Subtract4/2
  vo1/1 -> Subtract4/1, Subsystem1/1(in)
  Subtract1/1 -> Subtract2/1
  il1/1 -> Product/1
  Subsystem/1(x/s) -> Gain2/1  "Gamma"
  il/1 -> Subtract3/2
  delta1/1 -> Subsystem/2(x0)
  Subtract4/1 -> Gain5/1
  Gain5/1 -> Subtract6/2
  Gain4/1 -> Subtract5/2
  vo/1 -> Gain4/1
  Omega/1 -> Product/2
  Product/1 -> Gain3/1
  Gain3/1 -> Subtract2/2
  Gain2/1 -> Subtract1/2

== system WF_onshore/WT_MF2/Control System/Mechanical1 ==
  p : Inport
  pref : Inport  Port=2
  DeltaThetavsm0 : Inport  Port=3
  Omegavsm0 : Inport  Port=4
  Omegaref : Inport  Port=5
  Omegapll : Inport  Port=6
  Constant : Constant  Value=enable_pll
  Gain : Gain  Gain=1/cvtr.parameters.ta
  Gain1 : Gain  Gain=cvtr.parameters.kd
  Gain2 : Gain  Gain=cvtr.parameters.kdrpOmega
  Gain3 : Gain  Gain=cvtr.pu.Omegab
  Integrator1 : Integrator  InitialConditionSource=external
  Integrator2 : Integrator  InitialConditionSource=external
  Subtract : Sum  Inputs=-+--
  Subtract1 : Sum  Inputs=-+
  Subtract2 : Sum  Inputs=-+
  Switch : Switch  Criteria=u2 > Threshold  SaturateOnIntegerOverflow=off  InputSameDT=off
  Transfer Fcn (with initial outputs) : simulink_extras/Additional Linear/Transfer Fcn (with initial outputs)  N=[cvtr.parameters.Omegadf]  D="[1  cvtr.parameters.Omegadf]"  Y0=cvtr.ss.Kappa0  U0=cvtr.ss.Kappa0
  Thetavsm : Outport
  Omegavsm : Outport  Port=2
  wires:
  Integrator1/1 -> Thetavsm/1
  Switch/1 -> Subtract1/1
  Integrator2/1 -> Omegavsm/1, Subtract1/2, Subtract2/2, Transfer Fcn (with initial outputs)/1, Gain3/1
  Transfer Fcn (with initial outputs)/1 -> Switch/3
  Constant/1 -> Switch/2
  Omegapll/1 -> Switch/1
  Gain3/1 -> Integrator1/1
  Gain2/1 -> Subtract/4
  Subtract2/1 -> Gain2/1
  Omegaref/1 -> Subtract2/1
  Gain/1 -> Integrator2/1
  Omegavsm0/1 -> Integrator2/2
  Subtract1/1 -> Gain1/1
  Gain1/1 -> Subtract/3
  Subtract/1 -> Gain/1
  pref/1 -> Subtract/2
  p/1 -> Subtract/1
  DeltaThetavsm0/1 -> Integrator1/2

== system WF_onshore/WT_MF2/Control System/PLL1 ==
  note: DeltaOmegapll
  vo : Inport
  Add : Sum
  Add3 : Sum
  Constant : Constant  Value=cvtr.ss.Epsilonpll0
  Constant1 : Constant  Value=cvtr.ss.DeltaThetapll0
  Constant3 : Constant  Value=-cvtr.ss.DeltaThetapll0
  Constant4 : Constant  Value=cvtr.parameters.Omegan
  Demux : Demux  Outputs=2
  Demux1 : Demux  Outputs=2
  Gain : Gain  Gain=cvtr.parameters.kppll
  Gain1 : Gain  Gain=cvtr.pu.Omegab
  Gain2 : Gain  Gain=cvtr.parameters.kipll
  Integrator1 : Integrator  InitialConditionSource=external
  Integrator2 : Integrator  InitialConditionSource=external
  Multiport Switch1 : MultiPortSwitch  DataPortOrder=Zero-based contiguous  Inputs=2  zeroidx=on  SaturateOnIntegerOverflow=off  InputSameDT=off
  Mux : Mux  Inputs=2
  Subsystem1 : Subsystem
  Subsystem3 : Subsystem
  Terminator : Terminator
  Terminator1 : Terminator
  Transfer Fcn (with initial outputs) : simulink_extras/Additional Linear/Transfer Fcn (with initial outputs)  N=[cvtr.parameters.Omegalppll]  D="[1  cvtr.parameters.Omegalppll]"  Y0=real(cvtr.ss.vpll0)  U0=real(cvtr.ss.vpll0)
  Transfer Fcn (with initial outputs)1 : simulink_extras/Additional Linear/Transfer Fcn (with initial outputs)  N=[cvtr.parameters.Omegalppll]  D="[1  cvtr.parameters.Omegalppll]"  Y0=imag(cvtr.ss.vpll0)  U0=imag(cvtr.ss.vpll0)
  Trigonometric Function : Trigonometry  Operator=atan2
  delta6 : Constant  Value=selector_omega_reference
  Omegapll : Outport
  vpll : Outport  Port=2
  Thetapll : Outport  Port=3
  wires:
  Demux/2 -> Transfer Fcn (with initial outputs)1/1
  Multiport Switch1/1 -> Integrator1/2
  Constant1/1 -> Multiport Switch1/2
  delta6/1 -> Multiport Switch1/1
  Constant3/1 -> Multiport Switch1/3
  Integrator1/1 -> Thetapll/1
  Integrator2/1 -> Gain2/1
  Transfer Fcn (with initial outputs)/1 -> Trigonometric Function/2, Mux/1
  Demux/1 -> Transfer Fcn (with initial outputs)/1
  Demux1/1 -> Terminator/1  "vpll_d"
  Demux1/2 -> Terminator1/1  "vpll_q"
  Mux/1 -> Subsystem3/1(x_dq), Demux1/1
  Gain1/1 -> Integrator1/1
  Constant4/1 -> Add3/1
  Add3/1 -> Gain1/1, Omegapll/1
  Subsystem3/1(x_d+ix_q) -> vpll/1
  Add/1 -> Add3/2
  Gain2/1 -> Add/2
  Constant/1 -> Integrator2/2
  Gain/1 -> Add/1
  Trigonometric Function/1 -> Gain/1, Integrator2/1
  Transfer Fcn (with initial outputs)1/1 -> Mux/2, Trigonometric Function/1
  Subsystem1/1(x_dq) -> Demux/1
  vo/1 -> Subsystem1/1(x_d+ix_q)

== system WF_onshore/WT_MF2/Control System/PQ controller ==
  note: PI regulator
  note: PI regulator
  pref : Inport
  p : Inport  Port=2
  qref : Inport  Port=3
  q : Inport  Port=4
  Enable : EnablePort
  Gain : Gain  Gain=cvtr.parameters.kpp
  Gain1 : Gain  Gain=cvtr.parameters.kpq
  Gain2 : Gain  Gain=cvtr.parameters.kip
  Gain3 : Gain  Gain=cvtr.parameters.kiq
  Gain4 : Gain
  Gain5 : Gain  Gain=-1
  Integrator1 : Integrator  InitialConditionSource=external
  Integrator2 : Integrator  InitialConditionSource=external
  Mux : Mux  Inputs=2
  Subsystem3 : Subsystem
  Subtract1 : Sum  Inputs=|++
  Subtract2 : Sum  Inputs=|++
  Subtract3 : Sum  Inputs=|+-
  Subtract4 : Sum  Inputs=|+-
  delta1 : Constant  Value=cvtr.ss.GammaSd0
  delta2 : Constant  Value=cvtr.ss.GammaSq0
  ir : Outport
  wires:
  Gain4/1 -> Mux/1
  Gain5/1 -> Mux/2
  Subsystem3/1(x_d+ix_q) -> ir/1
  Subtract2/1 -> Gain5/1
  Subtract1/1 -> Gain4/1
  Mux/1 -> Subsystem3/1(x_dq)
  Gain1/1 -> Subtract2/1
  Integrator2/1 -> Gain3/1
  q/1 -> Subtract4/2
  Subtract4/1 -> Gain1/1, Integrator2/1
  delta2/1 -> Integrator2/2
  Gain3/1 -> Subtract2/2
  qref/1 -> Subtract4/1
  pref/1 -> Subtract3/1
  Gain2/1 -> Subtract1/2
  delta1/1 -> Integrator1/2
  Subtract3/1 -> Gain/1, Integrator1/1
  p/1 -> Subtract3/2
  Integrator1/1 -> Gain2/1
  Gain/1 -> Subtract1/1

== system WF_onshore/WT_MF2/Control System/Voltage controller DEM ==
  ve : Inport
  vo : Inport  Port=2
  Omegavsm : Inport  Port=3
  ilr0 : Inport  Port=4
  Enable : EnablePort
  Gain : Gain  Gain=cvtr.pu.Omegab/cvtr.parameters.ls
  Gain1 : Gain  Gain=cvtr.pu.Omegab/cvtr.parameters.ls
  Gain2 : Gain  Gain=cvtr.pu.Omegab*cvtr.parameters.rs/cvtr.parameters.ls
  Gain3 : Gain  Gain=1i*cvtr.pu.Omegab
  Product : Product  RndMeth=Zero
  Subsystem : Subsystem
  Subtract : Sum  Inputs=+---
  ilr : Outport
  wires:
  ilr0/1 -> Subsystem/2(x0)
  Subsystem/1(x/s) -> ilr/1, Gain2/1, Product/1
  ve/1 -> Gain/1
  Gain/1 -> Subtract/1
  vo/1 -> Gain1/1
  Gain1/1 -> Subtract/2
  Subtract/1 -> Subsystem/1(x)
  Gain2/1 -> Subtract/3
  Gain3/1 -> Subtract/4
  Product/1 -> Gain3/1
  Omegavsm/1 -> Product/2

== system WF_onshore/WT_MF2/Control System/Voltage controller QSEM ==
  ve : Inport
  vo : Inport  Port=2
  Omegavsm : Inport  Port=3
  Enable : EnablePort
  Constant : Constant  Value=cvtr.pu.Omegab*cvtr.parameters.rs/cvtr.parameters.ls
  Demux : Demux  Outputs=2
  Demux1 : Demux  Outputs=2
  Divide : Product  Inputs=*/
  Gain : Gain  Gain=cvtr.pu.Omegab/cvtr.parameters.ls
  Gain1 : Gain  Gain=cvtr.pu.Omegab/cvtr.parameters.ls
  Gain3 : Gain  Gain=1i*cvtr.pu.Omegab
  Mux : Mux  Inputs=2
  Subsystem2 : Subsystem
  Subsystem3 : Subsystem
  Subtract : Sum  Inputs=+-
  Subtract1 : Sum
  Terminator : Terminator
  Terminator1 : Terminator
  Transfer Fcn (with initial outputs) : simulink_extras/Additional Linear/Transfer Fcn (with initial outputs)  N=[cvtr.parameters.Omegavo]  D="[1  cvtr.parameters.Omegavo]"  Y0=cvtr.ss.vomd0  U0=cvtr.ss.vomd0
  Transfer Fcn (with initial outputs)1 : simulink_extras/Additional Linear/Transfer Fcn (with initial outputs)  N=[cvtr.parameters.Omegavo]  D="[1  cvtr.parameters.Omegavo]"  Y0=cvtr.ss.vomq0  U0=cvtr.ss.vomq0
  ilr : Outport
  wires:
  Transfer Fcn (with initial outputs)1/1 -> Mux/2
  Demux/2 -> Transfer Fcn (with initial outputs)1/1
  Demux/1 -> Transfer Fcn (with initial outputs)/1
  Demux1/2 -> Terminator1/1  "vomq?"
  Demux1/1 -> Terminator/1  "vomd?"
  Subsystem3/1(x_d+ix_q) -> Gain1/1
  Mux/1 -> Subsystem3/1(x_dq), Demux1/1
  Transfer Fcn (with initial outputs)/1 -> Mux/1
  Subsystem2/1(x_dq) -> Demux/1
  vo/1 -> Subsystem2/1(x_d+ix_q)
  Subtract1/1 -> Divide/2
  Divide/1 -> ilr/1
  Constant/1 -> Subtract1/1
  Subtract/1 -> Divide/1
  ve/1 -> Gain/1
  Gain/1 -> Subtract/1
  Gain1/1 -> Subtract/2
  Gain3/1 -> Subtract1/2
  Omegavsm/1 -> Gain3/1

== system WF_onshore/WT_MF2/Control System/Voltage controller VCVSM ==
  note: PI regulator
  note: Decoupling term
  note: Feedforward
  note: Voltage controller
  vo : Inport
  Omega : Inport  Port=2
  io : Inport  Port=3
  ve : Inport  Port=4
  Enable : EnablePort
  Gain : Gain  Gain=cvtr.parameters.kpv
  Gain1 : Gain  Gain=cvtr.parameters.rs
  Gain2 : Gain  Gain=cvtr.parameters.kiv
  Gain3 : Gain  Gain=1i*cvtr.parameters.cf
  Gain4 : Gain  Gain=cvtr.parameters.kffi
  Gain5 : Gain  Gain=1i*cvtr.parameters.ls
  Omega1 : InportShadow  Port=2
  Product : Product  RndMeth=Zero
  Product1 : Product
  Subsystem : Subsystem
  Subtract : Sum  Inputs=+--
  Subtract1 : Sum  Inputs=|++
  Subtract2 : Sum  Inputs=|++
  Subtract3 : Sum  Inputs=|+-
  Subtract5 : Sum  Inputs=|++
  delta1 : Constant  Value=cvtr.ss.Xi0
  io1 : InportShadow  Port=3
  vo1 : InportShadow
  ilr : Outport
  wires:
  Gain1/1 -> Subtract/2
  ve/1 -> Subtract/1
  Product1/1 -> Gain5/1
  Gain5/1 -> Subtract/3
  Omega1/1 -> Product1/2
  io1/1 -> Product1/1, Gain1/1
  Subtract5/1 -> ilr/1
  Subtract2/1 -> Subtract5/1
  Subtract1/1 -> Subtract2/1
  vo1/1 -> Product/1
  Subsystem/1(x/s) -> Gain2/1  "Xi"
  vo/1 -> Subtract3/2
  Subtract3/1 -> Subsystem/1(x), Gain/1
  delta1/1 -> Subsystem/2(x0)
  Gain4/1 -> Subtract5/2
  io/1 -> Gain4/1
  Omega/1 -> Product/2
  Product/1 -> Gain3/1
  Gain3/1 -> Subtract2/2
  Gain2/1 -> Subtract1/2
  Gain/1 -> Subtract1/1
  Subtract/1 -> Subtract3/1  "vor"

== system WF_onshore/WT_MF2/Control System/q droop1 ==
  q : Inport
  qref : Inport  Port=2
  vref : Inport  Port=3
  Gain3 : Gain  Gain=cvtr.parameters.kdrpq
  Subtract : Sum
  Subtract3 : Sum  Inputs=-+
  Transfer Fcn (with initial outputs) : simulink_extras/Additional Linear/Transfer Fcn (with initial outputs)  N=[cvtr.parameters.Omegaqf]  D="[1  cvtr.parameters.Omegaqf]"  Y0=cvtr.ss.q0  U0=cvtr.ss.q0
  ve : Outport
  qm : Outport  Port=2
  wires:
  q/1 -> Transfer Fcn (with initial outputs)/1
  Subtract/1 -> ve/1
  Gain3/1 -> Subtract/1
  Subtract3/1 -> Gain3/1
  Transfer Fcn (with initial outputs)/1 -> qm/1, Subtract3/1
  qref/1 -> Subtract3/2
  vref/1 -> Subtract/2

== system WF_onshore/WT_MF2/Transformations (pu and dq)/Park ==
  x_abc : Inport
  delta : Inport  Port=2
  Demux1 : Demux  Outputs=3
  Fcn : Fcn  Expr=2/3*(cos(u(4))*u(1)+cos(u(4)-2/3*pi)*u(2)+cos(u(4)+2/3*pi)*u(3))
  Fcn1 : Fcn  Expr=-2/3*(sin(u(4))*u(1)+sin(u(4)-2/3*pi)*u(2)+sin(u(4)+2/3*pi)*u(3))
  Mux : Mux
  Mux1 : Mux  Inputs=2
  x_dq : Outport
  wires:
  Mux1/1 -> x_dq/1
  Fcn1/1 -> Mux1/2
  Fcn/1 -> Mux1/1
  Mux/1 -> Fcn1/1, Fcn/1
  delta/1 -> Mux/4
  x_abc/1 -> Demux1/1
  Demux1/3 -> Mux/3
  Demux1/2 -> Mux/2
  Demux1/1 -> Mux/1

== system WF_onshore/WT_MF2/Transformations (pu and dq)/Park1 ==
  x_abc : Inport
  delta : Inport  Port=2
  Demux1 : Demux  Outputs=3
  Fcn : Fcn  Expr=2/3*(cos(u(4))*u(1)+cos(u(4)-2/3*pi)*u(2)+cos(u(4)+2/3*pi)*u(3))
  Fcn1 : Fcn  Expr=-2/3*(sin(u(4))*u(1)+sin(u(4)-2/3*pi)*u(2)+sin(u(4)+2/3*pi)*u(3))
  Mux : Mux
  Mux1 : Mux  Inputs=2
  x_dq : Outport
  wires:
  Demux1/1 -> Mux/1
  Demux1/2 -> Mux/2
  Demux1/3 -> Mux/3
  x_abc/1 -> Demux1/1
  delta/1 -> Mux/4
  Mux/1 -> Fcn/1, Fcn1/1
  Fcn/1 -> Mux1/1
  Fcn1/1 -> Mux1/2
  Mux1/1 -> x_dq/1

== system WF_onshore/WT_MF2/Transformations (pu and dq)/Park2 ==
  x_abc : Inport
  delta : Inport  Port=2
  Demux1 : Demux  Outputs=3
  Fcn : Fcn  Expr=2/3*(cos(u(4))*u(1)+cos(u(4)-2/3*pi)*u(2)+cos(u(4)+2/3*pi)*u(3))
  Fcn1 : Fcn  Expr=-2/3*(sin(u(4))*u(1)+sin(u(4)-2/3*pi)*u(2)+sin(u(4)+2/3*pi)*u(3))
  Mux : Mux
  Mux1 : Mux  Inputs=2
  x_dq : Outport
  wires:
  Demux1/1 -> Mux/1
  Demux1/2 -> Mux/2
  Demux1/3 -> Mux/3
  x_abc/1 -> Demux1/1
  delta/1 -> Mux/4
  Mux/1 -> Fcn/1, Fcn1/1
  Fcn/1 -> Mux1/1
  Fcn1/1 -> Mux1/2
  Mux1/1 -> x_dq/1

== system WF_onshore/WT_MF2/Transformations (pu and dq)/Park4 ==
  x_abc : Inport
  delta : Inport  Port=2
  Demux1 : Demux  Outputs=3
  Fcn : Fcn  Expr=2/3*(cos(u(4))*u(1)+cos(u(4)-2/3*pi)*u(2)+cos(u(4)+2/3*pi)*u(3))
  Fcn1 : Fcn  Expr=-2/3*(sin(u(4))*u(1)+sin(u(4)-2/3*pi)*u(2)+sin(u(4)+2/3*pi)*u(3))
  Mux : Mux
  Mux1 : Mux  Inputs=2
  x_dq : Outport
  wires:
  Demux1/1 -> Mux/1
  Demux1/2 -> Mux/2
  Demux1/3 -> Mux/3
  x_abc/1 -> Demux1/1
  delta/1 -> Mux/4
  Mux/1 -> Fcn/1, Fcn1/1
  Fcn/1 -> Mux1/1
  Fcn1/1 -> Mux1/2
  Mux1/1 -> x_dq/1

== system WF_onshore/WT_MF2/Transformations (pu and dq)/Subsystem2 ==
  x_dq : Inport
  Demux : Demux  Outputs=2
  Real-Imag to Complex : RealImagToComplex
  x_d+ix_q : Outport
  wires:
  Real-Imag to Complex/1 -> x_d+ix_q/1
  x_dq/1 -> Demux/1
  Demux/2 -> Real-Imag to Complex/2
  Demux/1 -> Real-Imag to Complex/1

== system WF_onshore/WT_MF2/Transformations (pu and dq)/Subsystem3 ==
  x_dq : Inport
  Demux : Demux  Outputs=2
  Real-Imag to Complex : RealImagToComplex
  x_d+ix_q : Outport
  wires:
  Real-Imag to Complex/1 -> x_d+ix_q/1
  x_dq/1 -> Demux/1
  Demux/2 -> Real-Imag to Complex/2
  Demux/1 -> Real-Imag to Complex/1

== system WF_onshore/WT_MF2/Transformations (pu and dq)/Subsystem4 ==
  x_dq : Inport
  Demux : Demux  Outputs=2
  Real-Imag to Complex : RealImagToComplex
  x_d+ix_q : Outport
  wires:
  Real-Imag to Complex/1 -> x_d+ix_q/1
  x_dq/1 -> Demux/1
  Demux/2 -> Real-Imag to Complex/2
  Demux/1 -> Real-Imag to Complex/1

== system WF_onshore/WT_MF2/Transformations (pu and dq)/Subsystem7 ==
  x_dq : Inport
  Demux : Demux  Outputs=2
  Real-Imag to Complex : RealImagToComplex
  x_d+ix_q : Outport
  wires:
  Demux/1 -> Real-Imag to Complex/1
  Demux/2 -> Real-Imag to Complex/2
  x_dq/1 -> Demux/1
  Real-Imag to Complex/1 -> x_d+ix_q/1

== system WF_onshore/WT_MF3/Control System/Current controller ==
  note: Active damping
  note: Feedforward
  note: Decoupling term
  note: PI regulator
  ilr : Inport
  il : Inport  Port=2
  Omega : Inport  Port=3
  vo : Inport  Port=4
  Gain : Gain  Gain=cvtr.parameters.kpc
  Gain1 : Gain
  Gain2 : Gain  Gain=cvtr.parameters.kic
  Gain3 : Gain  Gain=1i*cvtr.parameters.lf
  Gain4 : Gain  Gain=cvtr.parameters.kffv
  Gain5 : Gain  Gain=cvtr.parameters.kad
  Product : Product  RndMeth=Zero
  Subsystem : Subsystem
  Subsystem1 : Subsystem  mask{Omega=cvtr.parameters.Omegaad, xd0=cvtr.ss.Phid0, xq0=cvtr.ss.Phiq0}
  Subtract1 : Sum  Inputs=|++
  Subtract2 : Sum  Inputs=|++
  Subtract3 : Sum  Inputs=|+-
  Subtract4 : Sum  Inputs=|+-
  Subtract5 : Sum  Inputs=|++
  Subtract6 : Sum  Inputs=|+-
  delta1 : Constant  Value=cvtr.ss.Gamma0
  il1 : InportShadow  Port=2
  vo1 : InportShadow  Port=4
  vir : Outport
  wires:
  Gain2/1 -> Subtract1/2
  Gain3/1 -> Subtract2/2
  Product/1 -> Gain3/1
  Omega/1 -> Product/2
  vo/1 -> Gain4/1
  Gain4/1 -> Subtract5/2
  Gain5/1 -> Subtract6/2
  Subtract4/1 -> Gain5/1
  delta1/1 -> Subsystem/2(x0)
  il/1 -> Subtract3/2
  Subsystem/1(x/s) -> Gain2/1  "Gamma"
  il1/1 -> Product/1
  Subtract1/1 -> Subtract2/1
  vo1/1 -> Subsystem1/1(in), Subtract4/1
  Subsystem1/1(out) -> Subtract4/2
  Subtract2/1 -> Subtract5/1
  Subtract5/1 -> Subtract6/1
  Gain/1 -> Subtract1/1
  Subtract6/1 -> Gain1/1
  Gain1/1 -> vir/1
  Subtract3/1 -> Subsystem/1(x), Gain/1
  ilr/1 -> Subtract3/1
